simulink model "lookup_table_test"  (R2017b)
settings: Solver=VariableStepAuto  StartTime=0.0  StopTime=10.0  RelTol=1e-3
undefined symbols (not defined in the file): mtr_speed_rad, mtr_torque_Nm, opt_output_efficiency_location, opt_output_power_location, opt_output_torque_location
settings Model: Creator=Robert Wygant  LastModifiedBy=Robert Wygant

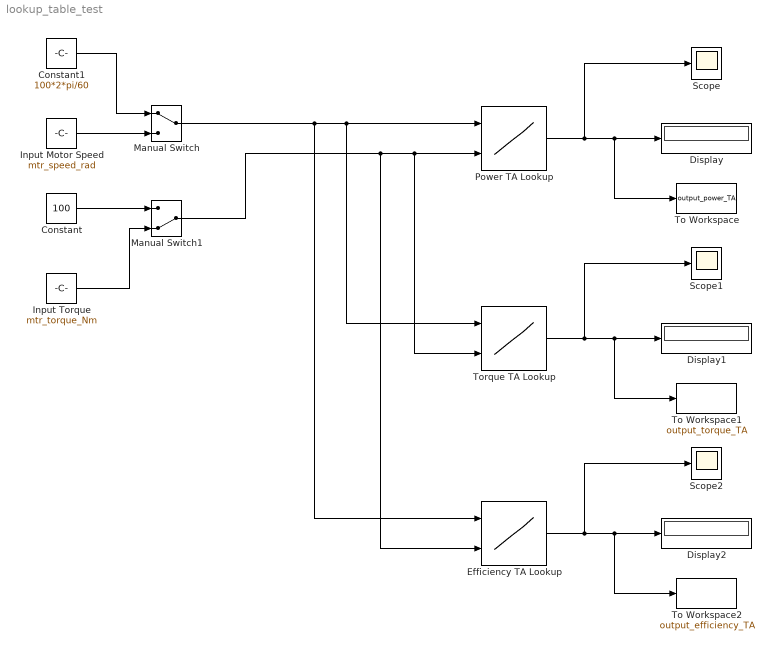
== system lookup_table_test ==
  Constant : Constant  Value=100
  Constant1 : Constant  Value=100*2*pi/60
  Display : Display
  Display1 : Display
  Display2 : Display
  Efficiency TA Lookup : Lookup_n-D  BreakpointsForDimension1=mtr_speed_rad  BreakpointsForDimension2=mtr_torque_Nm  Table=opt_output_efficiency_location  InternalRulePriority=Speed  RndMeth=Simplest  InputSameDT=on
  Input Motor Speed : Constant  Value=mtr_speed_rad
  Input Torque : Constant  Value=mtr_torque_Nm
  Manual Switch : ManualSwitch
  Manual Switch1 : ManualSwitch  CurrentSetting=0
  Power TA Lookup : Lookup_n-D  BreakpointsForDimension1=mtr_speed_rad  BreakpointsForDimension2=mtr_torque_Nm  Table=opt_output_power_location  InternalRulePriority=Speed  RndMeth=Simplest  InputSameDT=on
  Scope : Scope
  Scope1 : Scope
  Scope2 : Scope
  To Workspace : ToWorkspace  VariableName=output_power_TA  SampleTime=-1
      settings: Save2DSignal=2-D array (concatenate along first dimension)
  To Workspace1 : ToWorkspace  VariableName=output_torque_TA  SampleTime=-1
      settings: Save2DSignal=2-D array (concatenate along first dimension)
  To Workspace2 : ToWorkspace  VariableName=output_efficiency_TA  SampleTime=-1
      settings: Save2DSignal=2-D array (concatenate along first dimension)
  Torque TA Lookup : Lookup_n-D  BreakpointsForDimension1=mtr_speed_rad  BreakpointsForDimension2=mtr_torque_Nm  Table=opt_output_torque_location  InternalRulePriority=Speed  RndMeth=Simplest  InputSameDT=on
  wires:
  Power TA Lookup/1 -> Scope/1, To Workspace/1, Display/1
  Torque TA Lookup/1 -> Scope1/1, To Workspace1/1, Display1/1
  Efficiency TA Lookup/1 -> Scope2/1, To Workspace2/1, Display2/1
  Input Motor Speed/1 -> Manual Switch/2
  Manual Switch/1 -> Efficiency TA Lookup/1, Torque TA Lookup/1, Power TA Lookup/1
  Input Torque/1 -> Manual Switch1/2
  Constant/1 -> Manual Switch1/1
  Manual Switch1/1 -> Efficiency TA Lookup/2, Torque TA Lookup/2, Power TA Lookup/2
  Constant1/1 -> Manual Switch/1
